simulink model "measurments"  (R2014b)
settings: Solver=ode45  StartTime=0.0  StopTime=Time(end)  RelTol=1e-3
values from neighbouring files (symbols this model uses):
  rollGrad = 5*(pi/180)    (= 0.0872664625997)    [Init_for_washout_filter.m]    (also in Init_for_washout_filter2.m; Init_for_washout_filter3.m; Init_for_washout_filter4.m; UKF_start.m)
settings Model: Creator=eric  LastModifiedBy=eric

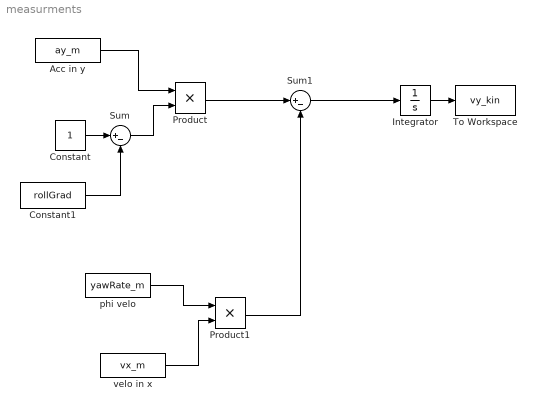
== system measurments ==
  Acc in y : FromWorkspace  VariableName=ay_m  SampleTime=0
  Constant : Constant
  Constant1 : Constant  Value=rollGrad
  Integrator : Integrator
  Product : Product
  Product1 : Product
  Sum : Sum  Inputs=|+-
  Sum1 : Sum  Inputs=|+-
  To Workspace : ToWorkspace  VariableName=vy_kin  SaveFormat=Timeseries  SampleTime=-1
  phi velo : FromWorkspace  VariableName=yawRate_m  SampleTime=0
  velo in x : FromWorkspace  VariableName=vx_m  SampleTime=0
  wires:
  Integrator/1 -> To Workspace/1
  Constant/1 -> Sum/1
  Constant1/1 -> Sum/2
  Sum/1 -> Product/2
  Acc in y/1 -> Product/1
  Product/1 -> Sum1/1
  Sum1/1 -> Integrator/1
  phi velo/1 -> Product1/1
  velo in x/1 -> Product1/2
  Product1/1 -> Sum1/2
